simulink model "Logic121"  (R2016b)
settings: Solver=VariableStepAuto  StartTime=0.0  StopTime=10.0  RelTol=1e-3
libraries: simulink x2
settings Model: Creator=viett  LastModifiedBy=viett

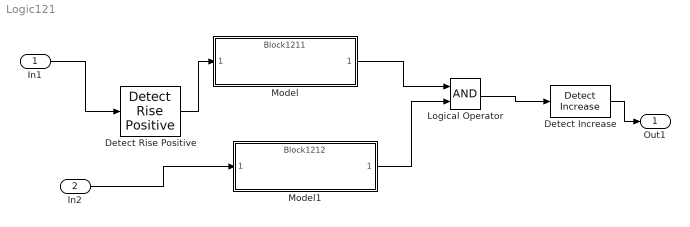
== system Logic121 ==
  In1 : Inport
  In2 : Inport  Port=2
  Detect Increase : simulink/Logic and Bit Operations/Detect Increase  vinit=0.0  OutDataTypeStr=boolean
  Detect Rise Positive : simulink/Logic and Bit Operations/Detect Rise Positive  vinit=0  OutDataTypeStr=boolean
  Logical Operator : Logic  AllPortsSameDT=off  OutDataTypeStr=boolean
  Model : ModelReference  ModelNameDialog=Block1211.slx  SimulationMode=Normal  ModelReferenceVersion=1.1
  Model1 : ModelReference  ModelNameDialog=Block1212.slx  SimulationMode=Normal  ModelReferenceVersion=1.1
  Out1 : Outport
  wires:
  Model1/1 -> Logical Operator/2
  Logical Operator/1 -> Detect Increase/1
  Model/1 -> Logical Operator/1
  Detect Rise Positive/1 -> Model/1
  In1/1 -> Detect Rise Positive/1
  In2/1 -> Model1/1
  Detect Increase/1 -> Out1/1
